simulink model "RobotX_ss_acousticsSKIP_dock_odoa_ta_1021"  (R2014a)
settings: Solver=FixedStepDiscrete  StartTime=0.0  StopTime=inf  FixedStep=.25  RelTol=1e-3
undefined symbols (not defined in the file): Com1, Com2, Com3, Com4, DiscIntNeverNeededParam, standard
libraries: xpcseriallib x42, simulink x8, slrtlib x8, speedgoatlib x2, speedgoatlib_IO102 x1
(part 16 of 19)

== matlab function RobotX_ss_acousticsSKIP_dock_odoa_ta_1021/Main FSM/ODOA/SLAM1/SLAM enabled/slammed ==
  data: mpa output; lm_data input; pre_part_positions input; part_positions output; positionboat input
%% SLAM by Chidananda Matada Shivananda
%  Copyright 2010 Randolph Voorhies

%  Edited 2014 Nick DiLeo - Modifications for unknown data association
%  and multiple measurements in a single timestep
    
%  Edited 2014 Chidananda Matada Shivananda - Simulink compatability, New
%  clustering technique added

%  This program is free software: you can redistribute it and/or modify
%  it under the terms of the GNU General Public License as published by
%  the Free Software Foundation, either version 3 of the License, or
%  (at your option) any later version.
%
%  This program is distributed in the hope that it will be useful,
%  but WITHOUT ANY WARRANTY; without even the implied warranty of
%  MERCHANTABILITY or FITNESS FOR A PARTICULAR PURPOSE.  See the
%  GNU General Public License for more details.
%
%  You should have received a copy of the GNU General Public License
%  along with this program.  If not, see <http://www.gnu.org/licenses/>.

function [mpa,part_positions]   = slammed(lm_data,pre_part_positions,positionboat)

%% General comments

% the angles in radians
% the ditance in m

%% Initialisations.

persistent particles avg_robot;
num_particles = 50;

% the limits
max_read_distance = 10;
min_read_distance = 5;
min_read_angle = -67.5*pi/180; %radians- maximum read angle
max_read_angle = 67.5*pi/180;

% The initial starting position of the robot Use UTM coordinates from GPS
avg_robot_position = [0;0;0];% x y rotation

% The Gaussian variance of the movement commands
% Approximating there are only two drives
% movement_variance = [.1;.1];   % Left drive Right_drive
% M = [movement_variance(1), 0.0;
%      0.0, movement_variance(2)];
measurement_variance = [0.01; 0.01];   % Distance Angle
R = [measurement_variance(1), 0.0;
    0.0, measurement_variance(2)];

default_importance=0.001;

if isempty(particles)
    %  Particles
    %             w[1]
    %             position[1,3]
    %             num_landmarks[300] this is to keep history
    
    %             lm_weight[2,15]based on number of landmarks
    %             landmarks[15]
    %                         position[2,1]
    %                         E[2,2]
    %                         counter[1]
    particles=repmat(struct('w',1.0/num_particles,'position',avg_robot_position,'num_landmarks',zeros(1,2),'lm_weight',repmat(1.0/num_particles,10,15),'landmarks',repmat(struct('pos',zeros(1,2),'E',zeros(2,2),'counter',0),1,15)),1,50);
    avg_robot_position = average_pos(particles,num_particles);
end

if isempty(avg_robot)
    avg_robot=avg_robot_position;
end

avg_robot_position=avg_robot;

%% Upload the moved data onto the particles
for shiva9=1:50
    particles(shiva9).position(1)= pre_part_positions(3*(shiva9-1)+1);
    particles(shiva9).position(2)= pre_part_positions(3*(shiva9-1)+1)*(pi/180);
    particles(shiva9).position(3)= pre_part_positions(3*(shiva9-1)+1);
end

%% Try to take a reading from each landmark and calculate the Jacobian
doResample = false;
% The input got from landmarks
[~,cols]=find(lm_data ~= 0);
if (isempty(cols)==0)% if the cols is not empty
    doResample=true; %if there is new measurement, then resample particles
end

if (doResample==true)
%     [r,~]=size(cols);
    [~,r]=size(cols);
    shiva=1;
    G=zeros(2,2,ceil(r/2));
    z_real=zeros(2,ceil(r/2));
    read_distance=zeros(ceil(r/2));
    read_angle=zeros(ceil(r/2));
    
    for lIdx = 1:2:r %amount of visible landmarks
        real_landmark = [lm_data(cols(lIdx+1)),lm_data(cols(lIdx))];
        % Take a real (noisy) measurement from the robot to the landmark
        %         [z_real(:,lIdx), G(:,:,lIdx)] = getRealMeasurement(avg_robot_position, real_landmark, [0 0]);
        %         function [z, H] = getRealMeasurement(pos, landmark_pos, observation_variance)
        
        landmark_angle=real_landmark(1);
        landmark_distance=real_landmark(2);
        % Compute the Jacobian of this measurement function
        q = landmark_distance^2.0;
        G(:,:,shiva) = [-(real_landmark(1) - avg_robot_position(1))/sqrt(q), -(real_landmark(2) - avg_robot_position(2))/sqrt(q);
            (real_landmark(2) - avg_robot_position(2))/q,       -(real_landmark(1) - avg_robot_position(1))/q];
        
        z_real(:,shiva) = [landmark_distance; landmark_angle];
        read_distance(shiva) = z_real(1,shiva);
        read_angle(shiva)    = z_real(2,shiva);
        shiva=shiva+1;
    end
    %     shiva=1;
    
    for pIdx = 1:num_particles
        %     particles(pIdx).lm_weight=[];
        %     clear z_p H Q
        %         coder.varsize('H', [2,2,16],[0 0 1]);
        num_landmarks=particles(pIdx).num_landmarks(1);
        assert(num_landmarks<20);
        H=zeros(2,2,num_landmarks);
        %         coder.varsize('z_p', [2 1 16]);
        z_p=zeros(2,1,num_landmarks);
        Q=zeros(2,2,num_landmarks);
        for j=1:particles(pIdx).num_landmarks(1)
            %             [z_p(:,j), H(:,:,j)] = getMeasurement(particles(pIdx).position, particles(pIdx).landmarks(j).pos, [0 0]);
            %             function [z, H] = getRealMeasurement(pos, landmark_pos, observation_variance)
            landmark_angle=particles(pIdx).landmarks(j).pos(1);
            landmark_distance=particles(pIdx).landmarks(j).pos(2);
            
            % Compute the Jacobian of this measurement function
            q = landmark_distance^2.0;
            %   H = [-(landmark_pos(1) - pos(1))/sqrt(q), -(landmark_pos(2) - pos(2))/sqrt(q), 0.0;
            %         (landmark_pos(2) - pos(2))/q,       -(landmark_pos(1) - pos(1))/q,      -1.0;
            %         0.0,                                0.0,                               1.0];
            
            H(:,:,j) = [-(particles(pIdx).landmarks(j).pos(1) - particles(pIdx).position(1))/sqrt(q), -(particles(pIdx).landmarks(j).pos(2) - particles(pIdx).position(2))/sqrt(q);
                (particles(pIdx).landmarks(j).pos(2) - particles(pIdx).position(2))/q,       -(particles(pIdx).landmarks(j).pos(1) - particles(pIdx).position(1))/q];
            
            
            z_p(:,j) = [landmark_distance;
                landmark_angle];
            
            for measured_lm=1:size(z_real,2)
                residual = z_real(:,measured_lm) - z_p(:,j);
                Q(:,:,j) = H(:,:,j)' * particles(pIdx).landmarks(j).E * H(:,:,j) + R;
                particles(pIdx).lm_weight(measured_lm,j) = particles(pIdx).w * norm(2*pi*Q(:,:,j)).^(-1/2)*exp(-1/2*(residual'/Q(:,:,j)*residual));
            end
        end
        
        particles(pIdx).num_landmarks(2)=particles(pIdx).num_landmarks(1);
        num_landmarks2=particles(pIdx).num_landmarks(2);
        assert(num_landmarks2<20);
        
        %           clear c_hat
        %         clear cost_table data_associate_mat data_associate_vect
        %%%%%%%%%%%%%%%%%%%%%%%%%%%%%%%%%%%%%%%%%%%%%%%%%%%%%%%%%%%%%%%%%%%%%%%%%%%%%%%%%%%%%%%%%%%%%%%%%%%%%%%%%%%%%%%%%%%%%%%%%%%%%%%%%%%%%%%%%%%%%
        cost_table=zeros(size(z_real,2),num_landmarks+size(z_real,2));
        %         cost_table=zeros(size(z_real,2),num_landmarks);
        
        if (num_landmarks~=0)
            cost_table(1:size(z_real,2),1:particles(pIdx).num_landmarks(1))=particles(pIdx).lm_weight(1:size(z_real,2),1:particles(pIdx).num_landmarks(1));
        end
        cost_table(1:size(z_real,2),particles(pIdx).num_landmarks(1)+1:particles(pIdx).num_landmarks(1)+size(z_real,2)) =default_importance*eye(size(z_real,2));
        
        particles(pIdx).w=max(max(cost_table,[],1),[],2);
        [~, idx_hold]=max(cost_table,[],1); %this is the max correseponding for each measurement
        for i=1:size(cost_table,2)
            idx_zero=setdiff(1:size(cost_table,1),idx_hold(i));
            cost_table(idx_zero,i)=0;
        end
        
        cost_table1=cost_table;
        for shiva14=1:size(cost_table,2)
            cost_table(:,shiva14)=cost_table1(:,size(cost_table,2)-shiva14+1);
        end
        
        
        new_landmarks=0;
        for measured_lm=1:size(z_real,2)
            [~, IDX] = max(cost_table(measured_lm,:));
            if IDX > particles(pIdx).num_landmarks(1)
                new_landmarks=new_landmarks+1;
            end
        end
        
        
        assert(new_landmarks<20);
        data_associate_mat=zeros(size(z_real,2),new_landmarks+num_landmarks2);
        
        for measured_lm=1:size(z_real,2)
            [~, IDX] = max(cost_table(measured_lm,:));
            if IDX > particles(pIdx).num_landmarks(1)
                %we haven't seen this landmark before
                %                 if particles(pIdx).num_landmarks(2)>14
                %                     break;
                %                 end
                particles(pIdx).num_landmarks(2)=particles(pIdx).num_landmarks(2)+1; %add new landmark
                data_associate_mat(measured_lm,particles(pIdx).num_landmarks(2))=measured_lm; %set correspondance b/t measurement and feature j
            else
                %we've already seen this landmark
                %           [val idx]=max(particles(pIdx).lm_weight(measured_lm,:));
                data_associate_mat(measured_lm,IDX)=measured_lm; %measurement is a known feature
            end
            
        end
        
        num_landmarks2=particles(pIdx).num_landmarks(2);
        assert(num_landmarks2<20);
        Hn=zeros(2,2,num_landmarks2);
        t=size(H);
        for i=1:t(3)
            Hn(:,:,i)=H(:,:,i);
        end
        
        %         H=zeros(2,2,num_landmarks2);
        H=Hn;
        
        data_associate_vect=max(data_associate_mat,[],1); %vector that contains measurement correspondance to landmarks
        i=1;
        feature_to_delete=zeros(num_landmarks2);
        for j=1:particles(pIdx).num_landmarks(2) %length(data_associate_vect)
            if (data_associate_vect(j)>0 && j>particles(pIdx).num_landmarks(1))
                % If we have never seen this landmark, then we need to initialize it.
                % We'll just use whatever first reading we recieved.
                particles(pIdx).landmarks(j).pos = [particles(pIdx).position(1) + ...
                    sin(read_angle(data_associate_vect(j))+particles(pIdx).position(3))*read_distance(data_associate_vect(j));...
                    particles(pIdx).position(2) + cos(read_angle(data_associate_vect(j))+particles(pIdx).position(3))*read_distance(data_associate_vect(j))]';
                % Initialize the landmark position covariance
                H(:,:,j)=G(:,:,data_associate_vect(j));
                particles(pIdx).landmarks(j).E = inv(G(:,:,data_associate_vect(j)))' * R * inv(G(:,:,data_associate_vect(j)));
                particles(pIdx).landmarks(j).counter=1; %initialize counter
            elseif (data_associate_vect(j)>0 && j<=particles(pIdx).num_landmarks(1))
                %we've seen this landmark before
                K = particles(pIdx).landmarks(j).E * H(:,:,j) / Q(:,:,j);
                % Mix the ideal reading, and our actual reading using the Kalman gain, and use the result
                % to predict a new landmark position
                particles(pIdx).landmarks(j).pos = particles(pIdx).landmarks(j).pos + (K*(z_real(:,data_associate_vect(j))-z_p(:,j)))';
                % Update the covariance of this landmark
                particles(pIdx).landmarks(j).E = (eye(size(H(:,:,j))) - K*H(:,:,j)')*particles(pIdx).landmarks(j).E;
                particles(pIdx).landmarks(j).counter=particles(pIdx).landmarks(j).counter+1; %increment counter
            else
                % We are leaving these unchanged.  These are commented
                % out, but this is what is actually happening in alg.
                % particles(pIdx).landmarks(j).pos = particles(pIdx).landmarks(j).pos;
                % particles(pIdx).landmarks(j).E=particles(pIdx).landmarks(j).E;
                dist_to_landmark=norm([particles(pIdx).landmarks(j).pos(1)-particles(pIdx).position(1) particles(pIdx).landmarks(j).pos(2)-particles(pIdx).position(2)]);
                ang_to_landmark=atan2((particles(pIdx).landmarks(j).pos(1) - particles(pIdx).position(1)),...
                    (particles(pIdx).landmarks(j).pos(2) - particles(pIdx).position(2)))-particles(pIdx).position(3);
                if (dist_to_landmark > max_read_distance ||dist_to_landmark < min_read_distance || ang_to_landmark > max_read_angle || ang_to_landmark < min_read_angle)
                    %counter(pIdx,j)=counter(pIdx,j) %don't change counter
                else
                    particles(pIdx).landmarks(j).counter=particles(pIdx).landmarks(j).counter-1; %decrement counter
                    if particles(pIdx).landmarks(j).counter<0
                        feature_to_delete(i)=j; %we're going to delete all these features at the end of the loop
                        i=i+1;
                    end
                end
                %
            end %if
        end %end j
        %     'pos',zeros(1,2),'E',zeros(2,2),'counter',0
        if~(isempty(nonzeros(feature_to_delete)))
            tobe_del=nonzeros(feature_to_delete);
            for shiva4=1:length(feature_to_delete)
                particles(pIdx).landmarks(tobe_del(shiva4)).pos=zeros(1,2);
                particles(pIdx).landmarks(tobe_del(shiva4)).E=zeros(2,2);
                particles(pIdx).landmarks(tobe_del(shiva4)).counter=0;
            end
            particles(pIdx).num_landmarks(2)= particles(pIdx).num_landmarks(2)-length(tobe_del);
        end
        
        particles(pIdx).num_landmarks(1)=particles(pIdx).num_landmarks(2);
        
    end %pIdx
    
    particles=resample(particles) ;
    
    
    
end% if (doResample==true)


%% Clustering
landmarks_positions=zeros(15*50,2);
row_counter=0;
for pIdx=1:num_particles
    for j=1:15 %this should be index timestep when in full script
        row_counter=row_counter+1;
        landmarks_positions(row_counter,:)=particles(pIdx).landmarks(j).pos(1:2)';
    end
end

[mpa,]=cluster(landmarks_positions,lm_data,positionboat);
max(landmarks_positions),max(mpa)
% 
% mpadi=mpa(:,1);
% mpaan=((mpa(:,2)));


%% new data prediction

%     lm_data_ind=lm_data(:)~=0;
%     lm_data_ind(1)=0;
%     lm_data1=lm_data(lm_data_ind);
%     
%     for j=(length(lm_data)/2)+1:(length(lm_data))
%         if lm_data(j)<91
%             lm_data(j)=psi(i)+lm_data(j);
%         else
%             lm_data(j)=psi(i)+lm_data(j)-360;
%         end
%     end
%     
%     if length(lm_data~=0)
%         x1=x(i)+(lm_data(1:length(lm_data)/2)/100).*sind(lm_data((length(lm_data)/2)+1:length(lm_data)));
%         y1=y(i)+(lm_data(1:length(lm_data)/2)/100).*cosd(lm_data((length(lm_data)/2)+1:length(lm_data)));
%     end

% landmarks_positions
% mpa1
% mpa=mpa1;




%% Final changes to be persistent
avg_robot=avg_robot_position;
part_positions=zeros(150,1);

for shiva9=1:3:150
    part_positions(shiva9)=particles(ceil(shiva9/3)).position(1);
    part_positions(shiva9+1)=(particles(ceil(shiva9/3)).position(2))*(180/pi);
    part_positions(shiva9+2)=particles(ceil(shiva9/3)).position(3);
end

%% Display and output

end %function [y,y1]  = slammed(imu_data,lm_data)

function [map,mapconv]= cluster(data,lm_add,positionboat)

n=size(data,1);
clusters=ones(n,1);
hubs=zeros(n,1);
hubs(1,1)=1;
dif=zeros(n,2);
% clustersort=zeros(n,3);
for i = 1:n
    dif(i,:)= data(clusters(i),:) - data(i,:);
end

dist =sum((dif.*dif),2);
counter =1;             %Keeps track of number of the present number of hubs
continue12 = 1;   % 1=true 0=false indicates whether to continue forming new
% rearr_lm(:,1)=lm_add(1:2:24)+rand(1);

while continue12
    counter = counter + 1;    % adding new hub
    if counter>750
        break;
    end
    [~,i]=max(dist);        %m= maximum value in the distance array
    %i is the location of the maximum value in the
    % array
    hubs(counter)=i;        %assigns index to new hub
    temp = i*ones(n,1);
    dif1=zeros(n,2);
    for i23 = 1:n
        dif1(i23,:)= data(temp(i23),:) - data(i23,:);
    end
    newdist =sum((dif1.*dif1),2);
    for r=1:n
        if newdist(r) < dist(r)
            dist(r)=newdist(r);
            clusters(r)=i;
        end     %end for if
    end
    maxdist=max(dist);      %returns distance of point farthest from its hub
    continue12 = farout(counter,hubs,data,maxdist); %Checks the stop condition
end

clustersort=[data,clusters];
clustersort=sortrows(clustersort,3);
map=zeros(12,2);
temp=zeros(12,1);
temp(1,1)=clustersort(1,3);
shiva12=1;
for i=1:n
    if sum(temp==clustersort(i,3)) == 0
        shiva12=shiva12+1;
        if shiva12>12
            break
        end
        temp(shiva12)=clustersort(i,3);
    end
end
for shiva13=1:12
    clusterIdx = clustersort(:,3)==temp(shiva13);
    map(shiva13,:)=[sum(clustersort(clusterIdx,1)),sum(clustersort(clusterIdx,2))]/(sum(clusterIdx)*50);
end
map(isnan(map))=0;

x=positionboat(1);
y=positionboat(2);
psi=positionboat(3);
for shiva17=1:2:23
    lm_add(shiva17+1)=lm_add(shiva17+1)*(180/pi);
    if lm_add(shiva17+1)<91
        lm_add(shiva17+1)=psi+lm_add(shiva17+1);
    else
        lm_add(shiva17+1)=psi+lm_add(shiva17+1)-360;
    end
end

shiva18=1;
mapconv=zeros(12,2);
for shiva17=1:2:23
    if (lm_add(shiva17)~=0 && lm_add(shiva17+1)~=0)
        mapconv(shiva18,1)=x+(lm_add(shiva17)*sind(lm_add(shiva17+1)));
        mapconv(shiva18,2)=y+(lm_add(shiva17)*cosd(lm_add(shiva17+1)));
        shiva18=shiva18+1;
    end
end

% map=map.*0.02;
for shiva19=1:12
   if (map(shiva19,1)<1000 && map(shiva19,1)~=0)
       map(shiva19,1)=map(shiva19,1)+4216.58; 
   end
   if (map(shiva19,2)<500 && map(shiva19,1)~=0)
       map(shiva19,2)=map(shiva19,2)+964; 
   end
end
% map(:,1)=map(:,1)+4216.58;
% map(:,2)=map(:,2)+964;
% map=map;
% map=map;
end

function continue1 = farout(counter1,hubs1,data1,maxdist1)

%FAROUT continue = farout(counter,hubs,data,maxdist)
%       Calculates stop condition.  Stops if the point farthest from its
%       hub is within the average distance value.

index1 = 0;
n=size(data1,1);
dif=zeros(n,2);
for i1 = 1:(counter1-1)
    for j = i1+1 : counter1
        index1 = index1 + 1;
        if index1>750
            break
        end
        dif(index1,:)=data1(hubs1(i1),:) - data1(hubs1(j),:);
    end
end

dist=sqrt(sum((dif.*dif),2));
average_dist = sum(dist)/(2*index1);
if (sqrt(maxdist1) < (average_dist/100000))
    continue1 = 0;
else continue1 =1;
end
end                             % end for farout

function avg_robot_position = average_pos(particles,num_particles)
xsiva=0;
ysiva=0;
rotasiva=0;

for siva=1:num_particles
    xsiva=xsiva+particles(siva).position(1);
    ysiva=ysiva+particles(siva).position(2);
    rotasiva=rotasiva+particles(siva).position(3);
end

avg_robot_position = [xsiva/num_particles; ysiva/num_particles; rotasiva/num_particles];

end

function [newParticles] = resample(oldParticles)
% Resample a group of particles such that those with higher weights have a
% higher chance of being replicated, and those with low weights have a high
% chance of disappearing
num_particles=50;
avg_robot_position = [0;0;0];% x y rotation
newParticles=repmat(struct('w',1.0/num_particles,'position',avg_robot_position,'num_landmarks',zeros(1,2),'lm_weight',repmat(1.0/num_particles,10,15),'landmarks',repmat(struct('pos',zeros(1,2),'E',zeros(2,2),'counter',0),1,15)),1,50);

weightSum = 0;
for i=1:length(oldParticles)
    weightSum = weightSum + oldParticles(i).w;
end
for i=1:length(oldParticles)
    oldParticles(i).w = oldParticles(i).w/weightSum;
end
M = length(oldParticles);
%   newParticles = [];
r = rand / M;
c = oldParticles(1).w;
i = 1;
shiva6=1;
assert(shiva6<51);
for m=1:M
    U = r + (m-1) * M^(-1);
    while U > c
        i = i+1;
        c = c+oldParticles(i).w;
    end
    newParticles(shiva6) = oldParticles(i);
    shiva6=shiva6+1;
end
for i=1:length(newParticles)
    newParticles(i).w = 1.0/length(newParticles);
end
end

== system RobotX_ss_acousticsSKIP_dock_odoa_ta_1021/Main FSM/ODOA/SLAM1/Models for prediction/Model7 ==
  X : Inport
  Y : Inport  Port=2
  Psi : Inport  Port=3
  Nav Messages : Inport  Port=4
  Bus Selector : BusSelector  OutputSignals=Velocity.u,Velocity.v,Velocity.r,Port.PtThrust,Port.PtAzimuth,Stbd.StThrust,Stbd.StAzimuth
  Data Store Read : DataStoreRead  DataStoreName=noiseLevel
  Demux : Demux  Outputs=3
  Discrete-Time Integrator1 : DiscreteIntegrator  SampleTime=-1  ICPrevOutput=DiscIntNeverNeededParam  ICPrevScaledInput=DiscIntNeverNeededParam
  Dynamic Model : MATLAB Function  TreatAsAtomicUnit=on
  Mux : Mux  Inputs=3
  Mux1 : Mux  Inputs=3
  Non-Holonomic Constraint : MATLAB Function  TreatAsAtomicUnit=on
  Port Thruster Model : MATLAB Function  TreatAsAtomicUnit=on
  Stbd Thruster Model : MATLAB Function  TreatAsAtomicUnit=on
  Sum : Sum  Inputs=|++|
  enabled : Constant
  move_part : MATLAB Function  TreatAsAtomicUnit=on
  NEyaw : Outport
  wires:
  Sum/1 -> Demux/1  "Forces"
  Bus Selector/2 -> Non-Holonomic Constraint/6(v), Dynamic Model/5(v)  "<v>"
  Bus Selector/1 -> Non-Holonomic Constraint/5(u), Dynamic Model/4(u)  "<u>"
  Psi/1 -> Non-Holonomic Constraint/8(psi), Dynamic Model/6(psi)
  Demux/2 -> Dynamic Model/2(F_sway)
  Demux/3 -> Dynamic Model/3(Torque)
  Demux/1 -> Dynamic Model/1(F_surge)
  Mux/1 -> Sum/2
  Stbd Thruster Model/1(F_surge) -> Mux/1
  Stbd Thruster Model/3(Torque) -> Mux/3
  Stbd Thruster Model/2(F_sway) -> Mux/2
  Mux1/1 -> Sum/1
  Port Thruster Model/2(F_sway) -> Mux1/2
  Port Thruster Model/1(F_surge) -> Mux1/1
  Port Thruster Model/3(Torque) -> Mux1/3
  Dynamic Model/1(surgeAccel) -> Non-Holonomic Constraint/2(surgeAccel)
  Dynamic Model/2(swayAccel) -> Non-Holonomic Constraint/3(swayAccel)
  Dynamic Model/3(yawAccel) -> Non-Holonomic Constraint/4(YawAccel)
  Y/1 -> Non-Holonomic Constraint/10(Y)
  X/1 -> Non-Holonomic Constraint/9(X)
  Bus Selector/3 -> Non-Holonomic Constraint/7(gyrz)  "<r>"
  Non-Holonomic Constraint/1(NEyaw) -> NEyaw/1
  enabled/1 -> Discrete-Time Integrator1/1
  Discrete-Time Integrator1/1 -> Non-Holonomic Constraint/1(time)
  Nav Messages/1 -> Bus Selector/1
  Bus Selector/4 -> move_part/1(PtThrust)  "<PtThrust>"
  Bus Selector/5 -> move_part/2(PtAzimuth)  "<PtAzimuth>"
  Bus Selector/7 -> move_part/4(StAzimuth)  "<StAzimuth>"
  Bus Selector/6 -> move_part/3(StThrust)  "<StThrust>"
  move_part/1(portMP) -> Port Thruster Model/1(portMP)
  move_part/2(portAzimuth) -> Port Thruster Model/2(portAzimuth)
  move_part/3(stbdMP) -> Stbd Thruster Model/1(stbdMP)
  move_part/4(stbdAzimuth) -> Stbd Thruster Model/2(stbdAzimuth)
  Data Store Read/1 -> move_part/5(noiseLevel)

== system RobotX_ss_acousticsSKIP_dock_odoa_ta_1021/Main FSM/ODOA/SLAM1/Models for prediction/Model8 ==
  X : Inport
  Y : Inport  Port=2
  Psi : Inport  Port=3
  Nav Messages : Inport  Port=4
  Bus Selector : BusSelector  OutputSignals=Velocity.u,Velocity.v,Velocity.r,Port.PtThrust,Port.PtAzimuth,Stbd.StThrust,Stbd.StAzimuth
  Data Store Read : DataStoreRead  DataStoreName=noiseLevel
  Demux : Demux  Outputs=3
  Discrete-Time Integrator1 : DiscreteIntegrator  SampleTime=-1  ICPrevOutput=DiscIntNeverNeededParam  ICPrevScaledInput=DiscIntNeverNeededParam
  Dynamic Model : MATLAB Function  TreatAsAtomicUnit=on
  Mux : Mux  Inputs=3
  Mux1 : Mux  Inputs=3
  Non-Holonomic Constraint : MATLAB Function  TreatAsAtomicUnit=on
  Port Thruster Model : MATLAB Function  TreatAsAtomicUnit=on
  Stbd Thruster Model : MATLAB Function  TreatAsAtomicUnit=on
  Sum : Sum  Inputs=|++|
  enabled : Constant
  move_part : MATLAB Function  TreatAsAtomicUnit=on
  NEyaw : Outport
  wires:
  Sum/1 -> Demux/1  "Forces"
  Bus Selector/2 -> Non-Holonomic Constraint/6(v), Dynamic Model/5(v)  "<v>"
  Bus Selector/1 -> Non-Holonomic Constraint/5(u), Dynamic Model/4(u)  "<u>"
  Psi/1 -> Non-Holonomic Constraint/8(psi), Dynamic Model/6(psi)
  Demux/2 -> Dynamic Model/2(F_sway)
  Demux/3 -> Dynamic Model/3(Torque)
  Demux/1 -> Dynamic Model/1(F_surge)
  Mux/1 -> Sum/2
  Stbd Thruster Model/1(F_surge) -> Mux/1
  Stbd Thruster Model/3(Torque) -> Mux/3
  Stbd Thruster Model/2(F_sway) -> Mux/2
  Mux1/1 -> Sum/1
  Port Thruster Model/2(F_sway) -> Mux1/2
  Port Thruster Model/1(F_surge) -> Mux1/1
  Port Thruster Model/3(Torque) -> Mux1/3
  Dynamic Model/1(surgeAccel) -> Non-Holonomic Constraint/2(surgeAccel)
  Dynamic Model/2(swayAccel) -> Non-Holonomic Constraint/3(swayAccel)
  Dynamic Model/3(yawAccel) -> Non-Holonomic Constraint/4(YawAccel)
  Y/1 -> Non-Holonomic Constraint/10(Y)
  X/1 -> Non-Holonomic Constraint/9(X)
  Bus Selector/3 -> Non-Holonomic Constraint/7(gyrz)  "<r>"
  Non-Holonomic Constraint/1(NEyaw) -> NEyaw/1
  enabled/1 -> Discrete-Time Integrator1/1
  Discrete-Time Integrator1/1 -> Non-Holonomic Constraint/1(time)
  Nav Messages/1 -> Bus Selector/1
  Bus Selector/4 -> move_part/1(PtThrust)  "<PtThrust>"
  Bus Selector/5 -> move_part/2(PtAzimuth)  "<PtAzimuth>"
  Bus Selector/7 -> move_part/4(StAzimuth)  "<StAzimuth>"
  Bus Selector/6 -> move_part/3(StThrust)  "<StThrust>"
  move_part/1(portMP) -> Port Thruster Model/1(portMP)
  move_part/2(portAzimuth) -> Port Thruster Model/2(portAzimuth)
  move_part/3(stbdMP) -> Stbd Thruster Model/1(stbdMP)
  move_part/4(stbdAzimuth) -> Stbd Thruster Model/2(stbdAzimuth)
  Data Store Read/1 -> move_part/5(noiseLevel)

== system RobotX_ss_acousticsSKIP_dock_odoa_ta_1021/Main FSM/ODOA/SLAM1/Models for prediction/Model9 ==
  X : Inport
  Y : Inport  Port=2
  Psi : Inport  Port=3
  Nav Messages : Inport  Port=4
  Bus Selector : BusSelector  OutputSignals=Velocity.u,Velocity.v,Velocity.r,Port.PtThrust,Port.PtAzimuth,Stbd.StThrust,Stbd.StAzimuth
  Data Store Read : DataStoreRead  DataStoreName=noiseLevel
  Demux : Demux  Outputs=3
  Discrete-Time Integrator1 : DiscreteIntegrator  SampleTime=-1  ICPrevOutput=DiscIntNeverNeededParam  ICPrevScaledInput=DiscIntNeverNeededParam
  Dynamic Model : MATLAB Function  TreatAsAtomicUnit=on
  Mux : Mux  Inputs=3
  Mux1 : Mux  Inputs=3
  Non-Holonomic Constraint : MATLAB Function  TreatAsAtomicUnit=on
  Port Thruster Model : MATLAB Function  TreatAsAtomicUnit=on
  Stbd Thruster Model : MATLAB Function  TreatAsAtomicUnit=on
  Sum : Sum  Inputs=|++|
  enabled : Constant
  move_part : MATLAB Function  TreatAsAtomicUnit=on
  NEyaw : Outport
  wires:
  Sum/1 -> Demux/1  "Forces"
  Bus Selector/2 -> Non-Holonomic Constraint/6(v), Dynamic Model/5(v)  "<v>"
  Bus Selector/1 -> Non-Holonomic Constraint/5(u), Dynamic Model/4(u)  "<u>"
  Psi/1 -> Non-Holonomic Constraint/8(psi), Dynamic Model/6(psi)
  Demux/2 -> Dynamic Model/2(F_sway)
  Demux/3 -> Dynamic Model/3(Torque)
  Demux/1 -> Dynamic Model/1(F_surge)
  Mux/1 -> Sum/2
  Stbd Thruster Model/1(F_surge) -> Mux/1
  Stbd Thruster Model/3(Torque) -> Mux/3
  Stbd Thruster Model/2(F_sway) -> Mux/2
  Mux1/1 -> Sum/1
  Port Thruster Model/2(F_sway) -> Mux1/2
  Port Thruster Model/1(F_surge) -> Mux1/1
  Port Thruster Model/3(Torque) -> Mux1/3
  Dynamic Model/1(surgeAccel) -> Non-Holonomic Constraint/2(surgeAccel)
  Dynamic Model/2(swayAccel) -> Non-Holonomic Constraint/3(swayAccel)
  Dynamic Model/3(yawAccel) -> Non-Holonomic Constraint/4(YawAccel)
  Y/1 -> Non-Holonomic Constraint/10(Y)
  X/1 -> Non-Holonomic Constraint/9(X)
  Bus Selector/3 -> Non-Holonomic Constraint/7(gyrz)  "<r>"
  Non-Holonomic Constraint/1(NEyaw) -> NEyaw/1
  enabled/1 -> Discrete-Time Integrator1/1
  Discrete-Time Integrator1/1 -> Non-Holonomic Constraint/1(time)
  Nav Messages/1 -> Bus Selector/1
  Bus Selector/4 -> move_part/1(PtThrust)  "<PtThrust>"
  Bus Selector/5 -> move_part/2(PtAzimuth)  "<PtAzimuth>"
  Bus Selector/7 -> move_part/4(StAzimuth)  "<StAzimuth>"
  Bus Selector/6 -> move_part/3(StThrust)  "<StThrust>"
  move_part/1(portMP) -> Port Thruster Model/1(portMP)
  move_part/2(portAzimuth) -> Port Thruster Model/2(portAzimuth)
  move_part/3(stbdMP) -> Stbd Thruster Model/1(stbdMP)
  move_part/4(stbdAzimuth) -> Stbd Thruster Model/2(stbdAzimuth)
  Data Store Read/1 -> move_part/5(noiseLevel)

== matlab function RobotX_ss_acousticsSKIP_dock_odoa_ta_1021/Main FSM/Termination/LLA to NED ==
  data: Course input; GoalLLA input; GoalNED output; NED_origin input
function GoalNED = LLA2NEDfun(Course,GoalLLA,NED_origin)
%Written by Anderson Lebbad on September 20, 2014
%Last edited by:
%
%This function converts a target Latitude, Longitude, Altitude (LLA) point
%into North, East, Down (NED) coordinates

%First convert to earth centered, earth fixed frame
GoalECEF1 = lla2ecef([GoalLLA(1,:)*(pi/180), 0]');
%Then convert from ECEF to North East Down
GoalNEDvect1 = ecef2ned(NED_origin'*(pi/180),GoalECEF1);
GoalNED1 = GoalNEDvect1(1:2)';

%First convert to earth centered, earth fixed frame
GoalECEF2 = lla2ecef([GoalLLA(2,:)*(pi/180), 0]');
%Then convert from ECEF to North East Down
GoalNEDvect2 = ecef2ned(NED_origin'*(pi/180),GoalECEF2);
GoalNED2 = GoalNEDvect2(1:2)';

GoalNED = (GoalNED1 + GoalNED2) / 2;

if Course == uint8('T')
    GoalNED = GoalLLA(1,:);
end

end

function x_ecef = lla2ecef(x_lla)
% LLE2ECEF: Converts from geodetic latitude, longitude, and altitude to earth-centered earth-fixed Cartesian coordinates
% INPUT: latitude phi (rad), longitude lambda (rad), altitude h (m)
% OUTPUT: [x, y, z]' (m) earth-centered earth-fixed Cartesian coordinates
    a = 6378137; % equatorial radius of ellipsoid (semi-major axis) (m)
    b = 6356752; % polar axis radius of ellipsoid (semi-minor axis) (m)

    phi = x_lla(1);
    lambda = x_lla(2);
    h = x_lla(3);
    
    % auxiliar quantities f, e, and N
    f = (a-b)/a;
    e = f*(2-f);
    N = a/sqrt(1-(e*sin(phi))^2);
    x_ecef = [(N+h)*cos(phi)*cos(lambda); (N+h)*cos(phi)*sin(lambda); (N*(1-e^2)+h)*sin(phi)];
end

function [x_ned] = ecef2ned(ned_lla, x_ecef)
% ECEF2NED Converts from earth-centered, earth-fixed Cartesian coordinates to tangent plane
% INPUT:
% 1) x_ecef=[x,y,z]' (m) earth-centered, earth-fixed Cartesian coordinates
% 2) ned_lla=[phi,lambda]' consiting of latitude phi (rad), longitude lambda (rad) of NED origin
% OUTPUT:
% 1) x_ned=[x,y,z]' (m) in NED coordinate system with the origin [phi,lambda]'

    phi = ned_lla(1);
    lambda = ned_lla(2);

    % transformation  matrix
    T = [-sin(phi)*cos(lambda) -sin(phi)*sin(lambda)  cos(phi)
         -sin(lambda)           cos(lambda)           0
          cos(phi)*cos(lambda)   cos(phi)*sin(lambda)  sin(phi)];

     x_ned = T*(x_ecef-lla2ecef([phi, lambda, 0]')); % convert to NED
     x_ned(3) = -x_ned(3);
end

== matlab function RobotX_ss_acousticsSKIP_dock_odoa_ta_1021/Main FSM/ODOA/GPS Move/CalcTimes ==
  data: pts input; u input; Data output
function Data = calcTimes(pts, u)
%Written by Anderson Lebbad on August 9, 2014
%Last Edited: Dylan DeGaetano September 1, 2014

%Calculates times for the boat to get to points for a trajectory, and
%formats Data for communication

%Initialize
Data = zeros(24,1);
traj = zeros(8,3);
traj(:,1:2) = pts;



for k = 2:8
    %Calculate distance to travel from last point
    distTravel = sqrt(sum((pts(k-1,:)-pts(k,:)).^2));
    %Assume 1m per second speed
    traj(k,3) = traj(k-1,3) + distTravel;
    %Add time based off initial velocity to get to first point past initial
    if k == 2
        traj(k,3) = traj(k,3) + 2.5*abs(2-u);
    end
end


%Output Data
for i=1:8
    for j = 1:3
        Data(3*(i-1)+j) = traj(i,j);
    end
end

== matlab function RobotX_ss_acousticsSKIP_dock_odoa_ta_1021/Sensors/1021 Comms/Lidar Send/MATLAB Function ==
  data: symbol input; LidarMode output; MainMode input
function LidarMode = selectLidarMode(symbol,MainMode)
%Written By Anderson Lebbad on October 21, 2014
%Last Edited By:
%
%This function decides the lidar mode to select based on the current task
%and docking symbol of the day.

if MainMode == 4
    LidarMode = symbol+2;
else
    LidarMode = 7;
end

end

== matlab function RobotX_ss_acousticsSKIP_dock_odoa_ta_1021/Main FSM/Start//Speedgate/Aim/LLA to NED ==
  data: LLA input; GoalNED output; NED_origin input
function GoalNED = LLA2NEDfun(LLA,NED_origin)
%Written by Anderson Lebbad on September 20, 2014
%Last edited by:
%
%This function converts a target Latitude, Longitude, Altitude (LLA) point
%into North, East, Down (NED) coordinates

%First convert to earth centered, earth fixed frame
GoalECEF = lla2ecef([LLA*(pi/180), 0]');
%Then convert from ECEF to North East Down
GoalNEDvect = ecef2ned(NED_origin'*(pi/180),GoalECEF);
GoalNED = GoalNEDvect(1:2)';


end

function x_ecef = lla2ecef(x_lla)
% LLE2ECEF: Converts from geodetic latitude, longitude, and altitude to earth-centered earth-fixed Cartesian coordinates
% INPUT: latitude phi (rad), longitude lambda (rad), altitude h (m)
% OUTPUT: [x, y, z]' (m) earth-centered earth-fixed Cartesian coordinates
    a = 6378137; % equatorial radius of ellipsoid (semi-major axis) (m)
    b = 6356752; % polar axis radius of ellipsoid (semi-minor axis) (m)

    phi = x_lla(1);
    lambda = x_lla(2);
    h = x_lla(3);
    
    % auxiliar quantities f, e, and N
    f = (a-b)/a;
    e = f*(2-f);
    N = a/sqrt(1-(e*sin(phi))^2);
    x_ecef = [(N+h)*cos(phi)*cos(lambda); (N+h)*cos(phi)*sin(lambda); (N*(1-e^2)+h)*sin(phi)];
end

function [x_ned] = ecef2ned(ned_lla, x_ecef)
% ECEF2NED Converts from earth-centered, earth-fixed Cartesian coordinates to tangent plane
% INPUT:
% 1) x_ecef=[x,y,z]' (m) earth-centered, earth-fixed Cartesian coordinates
% 2) ned_lla=[phi,lambda]' consiting of latitude phi (rad), longitude lambda (rad) of NED origin
% OUTPUT:
% 1) x_ned=[x,y,z]' (m) in NED coordinate system with the origin [phi,lambda]'

    phi = ned_lla(1);
    lambda = ned_lla(2);

    % transformation  matrix
    T = [-sin(phi)*cos(lambda) -sin(phi)*sin(lambda)  cos(phi)
         -sin(lambda)           cos(lambda)           0
          cos(phi)*cos(lambda)   cos(phi)*sin(lambda)  sin(phi)];

     x_ned = T*(x_ecef-lla2ecef([phi, lambda, 0]')); % convert to NED
     x_ned(3) = -x_ned(3);
end

== matlab function RobotX_ss_acousticsSKIP_dock_odoa_ta_1021/Sensors/1021 Comms/Message Selector/HRT Message/MATLAB Function ==
  data: Time input; asciiHRT output; HRTLat input; HRTLong input; HRTMode input; HRTTask input
% This function creates the heartbeat message to be sent from Speedgoat in
% ascii code
% Written by: Edward Zhu
% Date: 9/17/14

function asciiHRT = asciiHRTEncoder(Time, HRTLat, HRTLong, HRTMode, HRTTask)

% Initialize output message vector as the serial output block expects 128
% character message
asciiHRT = uint8(zeros(1,128));

% Convert static strings to ascii code
asciiHRTMsgID = uint8('$RXHRT,');
asciiComma = uint8(',');
asciiDeciPt = uint8('.');
if HRTLat >= 0
    asciiHRTNS = uint8('N,');
else
    HRTLat = -HRTLat;
    asciiHRTNS = uint8('S,');
end
if HRTLong >= 0
    asciiHRTEW = uint8('E,');
else
    HRTLong = -HRTLong;
    asciiHRTEW = uint8('W,');
end
asciiTeamID = uint8('FAUVU,');
asciiMsgEnd = uint8('*');
asciiMsgCRLF = [13 10];

% Convert UTC Time input (hhmmss) into ascii code
asciiTime = uint8(zeros(1,7));
asciiTime(7) = asciiComma;

for timeChar = 1:6
    asciiTime(timeChar) = floor(mod(Time,10^(7-timeChar))/...
        10^(6-timeChar)) + 48;
end

% Convert latitude (dd.mmmmmm) into ascii code
asciiHRTLat = uint8(zeros(1,10));
asciiHRTLat(10) = asciiComma;
asciiHRTLat(3) = asciiDeciPt;

HRTlatInt = floor(HRTLat);
for latIntChar = 1:2
    asciiHRTLat(latIntChar) = floor(mod(HRTlatInt,10^(3-latIntChar))/...
        10^(2-latIntChar)) + 48;
end

HRTlatDeci = mod(HRTLat,HRTlatInt) * 10^6;
for latDeciChar = 1:6
    asciiHRTLat(latDeciChar+3) = floor(mod(HRTlatDeci,10^(7-latDeciChar))/...
        10^(6-latDeciChar)) + 48;
end

% Convert longitude (ddd.mmmmmm) into ascii code
asciiHRTLong = uint8(zeros(1,11));
asciiHRTLong(11) = asciiComma;
asciiHRTLong(4) = asciiDeciPt;

HRTlongInt = floor(HRTLong);
for longIntChar = 1:3
    asciiHRTLong(longIntChar) = floor(mod(HRTlongInt,10^(4-longIntChar))/...
        10^(3-longIntChar)) + 48;
end

HRTlongDeci = mod(HRTLong,HRTlongInt) * 10^6;
for longDeciChar = 1:6
    asciiHRTLong(longDeciChar+4) = floor(mod(HRTlongDeci,10^(7-longDeciChar))/...
        10^(6-longDeciChar)) + 48;
end


% Convert vehicle mode into ascii (1 = RC, 2 = Auto)

HRTMode = HRTMode - 1; % LCM: RC = 2, Auto = 3
if HRTMode ~= 1 || 2
    HRTMode = 1;
    asciiHRTMode = [uint8(HRTMode+48) asciiComma];
else
    asciiHRTMode = [uint8(HRTMode+48) asciiComma];
end

% Convert vehicle task into ascii
HRTTask = HRTTask - 1; % FSM: Init = 1, SSGate = 2, SEA = 3, Dock = 4, LIT = 5, Obst = 6
if HRTTask ~= 1 || 2 || 3 || 4 || 5
    HRTTask = 1;
    asciiHRTTask = [uint8(HRTTask+48) asciiMsgEnd];
else
    asciiHRTTask = [uint8(HRTTask+48) asciiMsgEnd];
end

% Concat individual ascii arrays into one array
asciiHRTPreChkSum = cat(2,asciiHRTMsgID,asciiTime,asciiHRTLat,asciiHRTNS,asciiHRTLong,asciiHRTEW,...
    asciiTeamID,asciiHRTMode,asciiHRTTask);

% Calculate the checksum of the message from the '$' to the '*' and convert
% to hex
HRTchkSum = uint8(0);

for chksumChar = 1:(length(asciiHRTPreChkSum)-2)
    HRTchkSum = bitxor(HRTchkSum,asciiHRTPreChkSum(chksumChar+1));
end

% Convert the checksum to ascii
HRTchkSum = dec2hex(HRTchkSum);
asciiHRTChkSum = uint8(zeros(1,length(HRTchkSum))+32);
for i = 1:length(HRTchkSum)
    asciiHRTChkSum(i) = uint8(HRTchkSum(i));
end

% Concat the checksum and the '/r/n' to the end of the message
asciiHRTPostChkSum = cat(2,asciiHRTPreChkSum,asciiHRTChkSum,asciiMsgCRLF);

% Output the final message
asciiHRT(1:length(asciiHRTPostChkSum)) = asciiHRTPostChkSum;

== matlab function RobotX_ss_acousticsSKIP_dock_odoa_ta_1021/Sensors/1021 Comms/Message Selector/HRTLIT Message/MATLAB Function ==
  data: Time input; HRTLat input; HRTLong input; HRTTask input; HRTMode input; LITValid input; asciiHRTLIT output; LITSequence input
function asciiHRTLIT = asciiHRTLITEncoder(Time,HRTLat,HRTLong,HRTTask,HRTMode,LITValid,LITSequence)
% Initialize output message vector as the serial output block expects 128
% character message
asciiHRTLIT = uint8(zeros(1,128));

asciiComma = uint8(',');
asciiDeciPt = uint8('.');
asciiTeamID = uint8('FAUVU,');
asciiMsgEnd = uint8('*');
asciiMsgCRLF = [13 10];

% Convert UTC Time input (hhmmss) into ascii code
asciiTime = uint8(zeros(1,7));
asciiTime(7) = asciiComma;

for timeChar = 1:6
    asciiTime(timeChar) = floor(mod(Time,10^(7-timeChar))/...
        10^(6-timeChar)) + 48;
end

%%%%%%%%%%%%%%%%%%%%%%%%%%%%%%%%%%%%%%%%%%%%%%%%%%%%%%%%%%%%%%%%%%%%
% Heartbeat message
% Convert static strings to ascii code
asciiHRTMsgID = uint8('$RXHRT,');
if HRTLat >= 0
    asciiHRTNS = uint8('N,');
else
    HRTLat = -HRTLat;
    asciiHRTNS = uint8('S,');
end
if HRTLong >= 0
    asciiHRTEW = uint8('E,');
else
    HRTLong = -HRTLong;
    asciiHRTEW = uint8('W,');
end

% Convert latitude (dd.mmmmmm) into ascii code
asciiHRTLat = uint8(zeros(1,10));
asciiHRTLat(10) = asciiComma;
asciiHRTLat(3) = asciiDeciPt;

HRTlatInt = floor(HRTLat);
for latIntChar = 1:2
    asciiHRTLat(latIntChar) = floor(mod(HRTlatInt,10^(3-latIntChar))/...
        10^(2-latIntChar)) + 48;
end

HRTlatDeci = mod(HRTLat,HRTlatInt) * 10^6;
for latDeciChar = 1:6
    asciiHRTLat(latDeciChar+3) = floor(mod(HRTlatDeci,10^(7-latDeciChar))/...
        10^(6-latDeciChar)) + 48;
end

% Convert longitude (ddd.mmmmmm) into ascii code
asciiHRTLong = uint8(zeros(1,11));
asciiHRTLong(11) = asciiComma;
asciiHRTLong(4) = asciiDeciPt;

HRTlongInt = floor(HRTLong);
for longIntChar = 1:3
    asciiHRTLong(longIntChar) = floor(mod(HRTlongInt,10^(4-longIntChar))/...
        10^(3-longIntChar)) + 48;
end

HRTlongDeci = mod(HRTLong,HRTlongInt) * 10^6;
for longDeciChar = 1:6
    asciiHRTLong(longDeciChar+4) = floor(mod(HRTlongDeci,10^(7-longDeciChar))/...
        10^(6-longDeciChar)) + 48;
end

% Convert vehicle mode into ascii (1 = RC, 2 = Auto)
HRTMode = HRTMode - 1; % LCM: RC = 2, Auto = 3
if HRTMode ~= 1 || 2
    HRTMode = 1;
    asciiHRTMode = [uint8(HRTMode+48) asciiComma];
else
    asciiHRTMode = [uint8(HRTMode+48) asciiComma];
end

% Convert vehicle task into ascii
HRTTask = HRTTask - 1; % FSM: Init = 1, SSGate = 2, SEA = 3, Dock = 4, LIT = 5, Obst = 6
if HRTTask ~= 1 || 2 || 3 || 4 || 5
    HRTTask = 1;
    asciiHRTTask = [uint8(HRTTask+48) asciiMsgEnd];
else
    asciiHRTTask = [uint8(HRTTask+48) asciiMsgEnd];
end

% Concat individual ascii arrays into one array
asciiHRTPreChkSum = cat(2,asciiHRTMsgID,asciiTime,asciiHRTLat,asciiHRTNS,asciiHRTLong,asciiHRTEW,...
    asciiTeamID,asciiHRTMode,asciiHRTTask);

% Calculate the checksum of the message from the '$' to the '*' and convert
% to hex
HRTchkSum = uint8(0);

for chksumChar = 1:(length(asciiHRTPreChkSum)-2)
    HRTchkSum = bitxor(HRTchkSum,asciiHRTPreChkSum(chksumChar+1));
end

% Convert the checksum to ascii
HRTchkSum = dec2hex(HRTchkSum);
asciiHRTChkSum = uint8(zeros(1,length(HRTchkSum))+32);
for i = 1:length(HRTchkSum)
    asciiHRTChkSum(i) = uint8(HRTchkSum(i));
end

% Concat the checksum and the '/r/n' to the end of the message
asciiHRTPostChkSum = cat(2,asciiHRTPreChkSum,asciiHRTChkSum,asciiMsgCRLF);

%%%%%%%%%%%%%%%%%%%%%%%%%%%%%%%%%%%%%%%%%%%%%%%%%%%%%%%%%%%%%%%%%%%%%

% Light tower message
asciiLITMsgID = uint8('$RXLIT,');

% Convert the light sequece into ascii code (1 = R, 2 = B, 3 = G)
asciiLITSeq = uint8(zeros(1,4)+32);
asciiLITSeq(4) = asciiMsgEnd;

if LITValid == 1
    for seqChar = 1:3
        if LITSequence(seqChar) == 1
            LITSequence(seqChar) = uint8('R');
        elseif LITSequence(seqChar) == 2
            LITSequence(seqChar) = uint8('B');
        elseif LITSequence(seqChar) == 3
            LITSequence(seqChar) = uint8('G');
        end
    end
    asciiLITSeq(1:3) = LITSequence;
end

% Concat individual ascii arrays into one array
asciiLITPreChkSum = cat(2,asciiLITMsgID,asciiTime,asciiTeamID,asciiLITSeq);

% Calculate the checksum of the message from the '$' to the '*' and convert
% to hex
LITchkSum = uint8(0);

for chksumChar = 1:(length(asciiLITPreChkSum)-2)
    LITchkSum = bitxor(LITchkSum,asciiLITPreChkSum(chksumChar+1));
end

% Convert the checksum to ascii
LITchkSum = dec2hex(LITchkSum);
asciiLITChkSum = uint8(zeros(1,length(LITchkSum))+32);
for i = 1:length(LITchkSum)
    asciiLITChkSum(i) = uint8(LITchkSum(i));
end

% Concat the checksum and the '/r/n' to the end of the message
asciiLITPostChkSum = cat(2,asciiLITPreChkSum,asciiLITChkSum,asciiMsgCRLF);

%%%%%%%%%%%%%%%%%%%%%%%%%%%%%%%%%%%%%%%%%%%%%%%%%%%%%%%%%%%%%%%%%%%%%%%%%%%

asciiHRTLITPostChkSum = cat(2,asciiHRTPostChkSum,asciiLITPostChkSum);
asciiHRTLIT(1:length(asciiHRTLITPostChkSum)) = asciiHRTLITPostChkSum;

== matlab function RobotX_ss_acousticsSKIP_dock_odoa_ta_1021/Main FSM/Aim/MATLAB Function ==
  data: ssHeldHeading input; X input; Data output; Y input
function Data  = Orient(ssHeldHeading, X, Y)
%Written by Dylan DeGaetano on September 2, 2014
%Last Edited:Dylan DeGaetano on September 10,2014

%This function passes the current pose data added to the angle of the Light 
%buoy This stare forces the Boat to stare at the bouy.This task must be in station 
%keeping mode

persistent holdPose

if isempty(holdPose)
    holdPose = [X, Y, ssHeldHeading];
end

%Initialize Data variable
Data = zeros(24,1);

%Set desired pose
Data(1) = holdPose(1);
Data(2) = holdPose(2);
Data(3) = holdPose(3);

end

== matlab function RobotX_ss_acousticsSKIP_dock_odoa_ta_1021/Main FSM/ODOA/GPS Move/GPSMove ==
  data: GoalNED input; X input; Finished output; valid output; Y input; Psi input; pts output
function [Finished,valid,pts] = GPSmove(GoalNED,X,Y,Psi)
%Written by Dylan DeGaetano on September 1, 2014
%Last edited by: Anderson Lebbad
%
%This function will go to a given NED cooridnate, last edit changed the
%goal pt and variable names

persistent Sample
if isempty(Sample)
Sample = 0;
end
Finished = 0;
pts = zeros(8,2);
%$Distance to object in meters
if Sample == 100
    Sample = 0;
end

if Sample == 0
    pts(1,1) = X+5*cos(Psi*pi/180);
    pts(1,2) = Y+5*sin(Psi*pi/180);
    pts(8,1) = GoalNED(1,1);
    pts(8,2) = GoalNED(1,2);
    pts(2,:) = pts(1,:) +(1*(GoalNED-pts(1,:))/7);
    pts(3,:) = pts(1,:) +(2*(GoalNED-pts(1,:))/7);
    pts(4,:) = pts(1,:) +(3*(GoalNED-pts(1,:))/7);
    pts(5,:) = pts(1,:) +(4*(GoalNED-pts(1,:))/7);
    pts(6,:) = pts(1,:) +(5*(GoalNED-pts(1,:))/7);
    pts(7,:) = pts(1,:) +(6*(GoalNED-pts(1,:))/7);
    Sample = 1; 
    valid = 1;
    
else 
    range = sqrt(sum((GoalNED - [X Y]).^2));
    if range <= 5
        Finished = 1;
    end
    valid = 0;
    Sample = Sample + 1;
end

== matlab function RobotX_ss_acousticsSKIP_dock_odoa_ta_1021/Main FSM/Start//Speedgate/GPS Move/CalcTimes ==
  data: pts input; u input; Data output
function Data = calcTimes(pts, u)
%Written by Anderson Lebbad on August 9, 2014
%Last Edited: Dylan DeGaetano September 1, 2014

%Calculates times for the boat to get to points for a trajectory, and
%formats Data for communication

%Initialize
Data = zeros(24,1);
traj = zeros(8,3);
traj(:,1:2) = pts;



for k = 2:8
    %Calculate distance to travel from last point
    distTravel = sqrt(sum((pts(k-1,:)-pts(k,:)).^2));
    %Assume 1m per second speed
    traj(k,3) = traj(k-1,3) + distTravel;
    %Add time based off initial velocity to get to first point past initial
    if k == 2
        traj(k,3) = traj(k,3) + 2.5*abs(2-u);
    end
end


%Output Data
for i=1:8
    for j = 1:3
        Data(3*(i-1)+j) = traj(i,j);
    end
end

== matlab function RobotX_ss_acousticsSKIP_dock_odoa_ta_1021/Main FSM/Start//Speedgate/GPS Move/GPSMove ==
  data: GoalNED input; X input; Finished output; valid output; Y input; Psi input; pts output
function [Finished,valid,pts] = GPSmove(GoalNED,X,Y,Psi)
%Written by Dylan DeGaetano on September 1, 2014
%Last edited by: Anderson Lebbad
%
%This function will go to a given NED cooridnate, last edit changed the
%goal pt and variable names

persistent Sample
if isempty(Sample)
Sample = 0;
end
Finished = 0;
pts = zeros(8,2);
%$Distance to object in meters
if Sample >= 100
    Sample = 0;
end

if Sample == 0
    pts(1,1) = X+5*cos(Psi*pi/180);
    pts(1,2) = Y+5*sin(Psi*pi/180);
    pts(8,1) = GoalNED(1,1);
    pts(8,2) = GoalNED(1,2);
    pts(2,:) = pts(1,:) +(1*(GoalNED-pts(1,:))/7);
    pts(3,:) = pts(1,:) +(2*(GoalNED-pts(1,:))/7);
    pts(4,:) = pts(1,:) +(3*(GoalNED-pts(1,:))/7);
    pts(5,:) = pts(1,:) +(4*(GoalNED-pts(1,:))/7);
    pts(6,:) = pts(1,:) +(5*(GoalNED-pts(1,:))/7);
    pts(7,:) = pts(1,:) +(6*(GoalNED-pts(1,:))/7);
    Sample = 1; 
    valid = 1;
    
else 
    range = sqrt(sum((GoalNED - [X Y]).^2));
    if range <= 8
        Finished = 1;
    end
    valid = 0;
    Sample = Sample + 1;
end

== matlab function RobotX_ss_acousticsSKIP_dock_odoa_ta_1021/Main FSM/Start//Speedgate/Main Enabler ==
  data: taskSelector output; GpsEn output; entEn output; exitEn output; ssgateTask input; GpsFin input; entFin input
function [taskSelector,GpsEn,entEn,exitEn]=Startgate_Enabler(ssgateTask,...
    GpsFin,entFin)
%Written by Anderson Lebbad on July 19, 2013
%Last Edited: Dylan DeGaetano on September ,4 2014
%   Substring search for task was written in
%   Case switches were redundant, combined with first set of if statements

%Changes the value of MainMode and the enablers for the tasks within the
%Main FSM.

% Initialize enable signals
GpsEn = 0;
entEn =0;
exitEn = 0;

% Convert main task indicator to a string
ssgateTaskStr = char(ssgateTask);

% Adjust finished states based on user task selection (never skips
% initialization)
if ~isempty(strfind(ssgateTaskStr,'Aim'))
    GpsFin = 1;
elseif ~isempty(strfind(ssgateTaskStr,'Start'))
    GpsFin = 1;
    entFin = 1;
elseif ~isempty(strfind(ssgateTaskStr,'Speed'))
    GpsFin = 1;
    entFin = 1;
end

% Set enable signals based on state completion
if GpsFin == 0
    GpsEn = 1;
    taskSelector = 1;
elseif entFin == 0
    entEn = 1;
    taskSelector = 2;
else
    exitEn = 1;
    taskSelector = 3;
end

== matlab function RobotX_ss_acousticsSKIP_dock_odoa_ta_1021/Main FSM/ODOA/ODOA Enabler ==
  data: taskSelector output; GpsEn output; PathEn output; mainTask input; GpsFin input
function [taskSelector,GpsEn,PathEn]=ODOA_Enabler(mainTask,GpsFin)
%Written by Anderson Lebbad on July 19, 2013
%Last Edited: Dylan DeGaetano on September ,4 2014
%   Substring search for task was written in
%   Case switches were redundant, combined with first set of if statements

%Changes the value of MainMode and the enablers for the tasks within the
%Main FSM.

% Initialize enable signals
GpsEn = 0;
PathEn = 0;

% Convert main task indicator to a string
mainTaskStr = char(mainTask);

% Adjust finished states based on user task selection (never skips
% initialization)
if ~isempty(strfind(mainTaskStr,'Path'))
    GpsFin = 1;
end

% Set enable signals based on state completion
if GpsFin == 0
    GpsEn = 1;
    taskSelector = 1;
else
    PathEn = 1 ;
    taskSelector = 2;
end
